simulink model "IntegratedBehaviorModule"  (R2024b)
settings: Solver=VariableStepAuto  StartTime=0.0  StopTime=inf  RelTol=1e-3
StartFcn:
  | clf
model workspace (MAT data in the model file):
  SL_ROS_VariableLengthArrays_MaxSizes.CommonInfo.ArrayTruncateAction = 'EmitWarning'
  SL_ROS_VariableLengthArrays_MaxSizes.MsgTypeMap = containers.Map
  SL_ROS_VariableLengthArrays_MaxSizes.MsgTypeMap.serialization.keys = {'std_msgs/Float32MultiArray', 'std_msgs/Float64MultiArray', 'std_msgs/Int8MultiArray'}
  SL_ROS_VariableLengthArrays_MaxSizes.MsgTypeMap.serialization.values{1}.PropertyName = 'data'
  SL_ROS_VariableLengthArrays_MaxSizes.MsgTypeMap.serialization.values{1}.DataType = 'single'
  SL_ROS_VariableLengthArrays_MaxSizes.MsgTypeMap.serialization.values{1}.MaxLength = 1500000
  SL_ROS_VariableLengthArrays_MaxSizes.MsgTypeMap.serialization.values{2}.PropertyName = 'data'
  SL_ROS_VariableLengthArrays_MaxSizes.MsgTypeMap.serialization.values{2}.DataType = 'double'
  SL_ROS_VariableLengthArrays_MaxSizes.MsgTypeMap.serialization.values{2}.MaxLength = 1500000
  SL_ROS_VariableLengthArrays_MaxSizes.MsgTypeMap.serialization.values{3}.PropertyName = 'data'
  SL_ROS_VariableLengthArrays_MaxSizes.MsgTypeMap.serialization.values{3}.DataType = 'int8'
  SL_ROS_VariableLengthArrays_MaxSizes.MsgTypeMap.serialization.values{3}.MaxLength = 1500000
  SL_ROS_VariableLengthArrays_MaxSizes.MsgTypeMap.serialization.uniformity = 0
  SL_ROS_VariableLengthArrays_MaxSizes.MsgTypeMap.serialization.keyType = 'char'
  SL_ROS_VariableLengthArrays_MaxSizes.MsgTypeMap.serialization.valueType = 'any'
  Sig = Simulink.Signal
  Sig.Dimensions = -1
  Sig.DimensionsMode = 'auto'
  Sig.Complexity = 'auto'
  Sig.SampleTime = -1
  Sig.SamplingMode = 'auto'
  Sig.DataType = 'auto'
undefined symbols (not defined in the file or in its folder): dem, fixedTEBParams, goalPose, initialTranslationTruck, mapSize, maxRefPathLen, nlobjTracking, pathBus_struct, TaskControllerModeType, tuneableTEBParamsCpp, tuneableTerrainAwareParams, worldGridLoc, worldMat, worldRes
libraries: simulink x10, roshelperlib x5, robotmobilelib x1, robotsim3dlib x1, sim3dlib x1
(part 1 of 2)
settings Model: DataDictionary=ros2lib.sldd  Creator=cstabile  LastModifiedBy=jbrault
settings SolverCC: DateTimeAtSimulationTimeZero=[]
settings OptimizationCC: BlockReduction=off  EnhancedBackFolding=on  PassReuseOutputArgsAs=Individual arguments  ZeroExternalMemoryAtStartup=off  ZeroInternalMemoryAtStartup=off  MaxStackSize=64  OptimizeBlockOrder=speed  DifferentSizesBufferReuse=on  OptimizationCustomize=off  EfficientTunableParamExpr=on
settings DebuggingCC: ParameterTunabilityLossMsg=error
settings ModelReferenceCC: UpdateModelReferenceTargets=IfOutOfDate
settings SFSimCC: SimTargetLang=C++
settings RTWCC: Description=Embedded Coder  SystemTargetFile=ert.tlc  HardwareBoard=Robot Operating System 2 (ROS 2)  TLCOptions="-aInlineSetEventsForThisBaseRateFcn=TLC_FALSE -aSuppressMultiTaskScheduler=TLC_FALSE  -aRateBasedStepFcn=0"  TemplateMakefile=ert_default_tmf  Toolchain=Colcon Tools  TargetLang=C++  GPUComputeCapability=3.5
settings CodeAppCC: ForceParamTrailComments=on  IgnoreCustomStorageClasses=off  OperatorAnnotations=on  SimulinkDataObjDesc=on  SFDataObjDesc=on  InsertBlockDesc=on
settings ERTTargetCC: CodeInterfacePackaging=C++ class  InlinedParameterPlacement=Hierarchical  RootIOFormat=Structure reference  DynamicArrayContainerType=coder::array

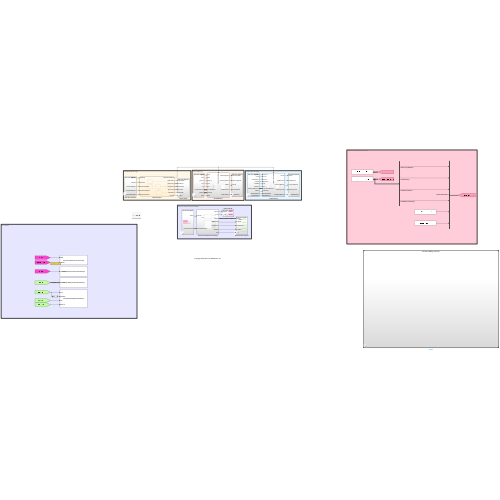
[thumbnail: Simulink's stored preview of the top-level diagram]
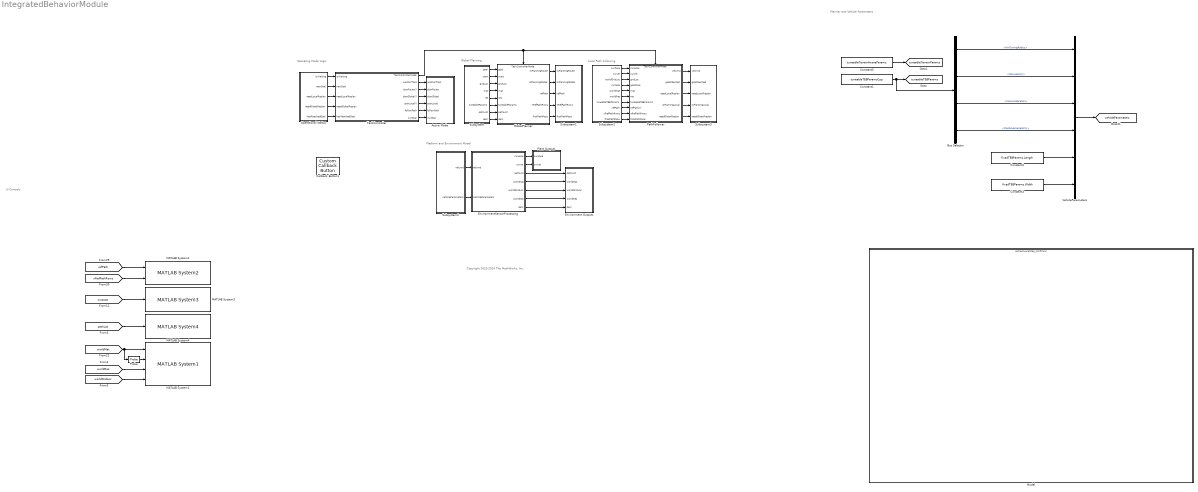
== system IntegratedBehaviorModule ==
  note: UI Controls
  note: Local Path Following
  note: Planner and Vehicle Parameters
  note: Global Planning
  note: Platform and Enviornment Model
  note: Operating Mode Logic
  note: Copyright 2023-2024 The MathWorks, Inc.
  Active Mode : Subsystem  Variant=on  VariantControl=Subsystem7
  Bus Selector : BusSelector  OutputSignals=MinTurningRadius,MaxVelocity,MaxAcceleration,MaxReverseVelocity
  Callback Button1 : CustomCallbackButton  Configuration="{\"components\":[{\"name\":\"BackgroundImageComponent\",\"settings\":{\"image\":{\"size\":[0,0],\"src\":\"default\",\"srcOrientation\":\"Right\"},\"position\":[0,0,1,1]}},{\"name\":\"ButtonStateComponent\",\"settings\":{\"buttonType\":\"momentary\",\"clickFcn\":\"set_param([bdroot(gcb) '\\/Operational Status\\/Simulink Signals\\/Confirm New Goal\\/newGoalBlock'],'Value','goalPose');\",\"onValue\":1,\"position\":[0,0,1,1],\"pressDelay\":\"500\",\"pressFcn\":\"\",\"repeatInterval\":\"0\",\"states\":[{\"horizontalAlignment\":\"center\",\"image\":{\"position\":[0,0,1,1],\"size\":[1,1],\"src\":\"default\",\"srcOrientation\":\"Right\"},\"label\":{\"color\":[0.01176470588,0.01176470588,0.01176470588,1],\"icon\":{\"size\":[0,0],\"src\":\"default\",\"srcOrientation\":\"Right\"},\"iconPlacement\":\"left\",\"opacity\":1,\"show\":true,\"text\":{\"content\":\"Update Goal\",\"font\":\"Helvetica\"}},\"labelOffset\":[0,0],\"verticalAlignment\":\"middle\"},{\"horizontalAlignment\":\"center\",\"image\":{\"position\":[0,0,1,1],\"size\":[1,1],\"src\":\"default\",\"srcOrientation\":\"Right\"},\"label\":{\"color\":[0.01176470588,0.01176470588,0.01176470588,1],\"icon\":{\"size\":[0,0],\"src\":\"default\",\"srcOrientation\":\"Right\"},\"iconPlacement\":\"left\",\"opacity\":1,\"show\":true,\"text\":{\"content\":\"Update Goal\",\"font\":\"Helvetica\"}},\"labelOffset\":[0,0],\"verticalAlignment\":\"middle\"},{\"horizontalAlignment\":\"center\",\"image\":{\"position\":[0,0,1,1],\"size\":[1,1],\"src\":\"default\",\"srcOrientation\":\"Right\"},\"label\":{\"color\":[0.01176470588,0.01176470588,0.01176470588,1],\"icon\":{\"size\":[0,0],\"src\":\"default\",\"srcOrientation\":\"Right\"},\"iconPlacement\":\"left\",\"opacity\":1,\"show\":true,\"text\":{\"content\":\"Update Goal\",\"font\":\"Helvetica\"}},\"labelOffset\":[0,0],\"verticalAlignment\":\"middle\"},{\"horizontalAlignment\":\"center\",\"image\":{\"position\":[0,0,1,1],\"size\":[1,1],\"src\":\"default\",\"srcOrientation\":\"Right\"},\"label\":{\"color\":[0.01176470588,0.01176470588,0.01176470588,1],\"icon\":{\"size\":[0,0],\"src\":\"default\",\"srcOrientation\":\"Right\"},\"iconPlacement\":\"left\",\"opacity\":1,\"show\":true,\"text\":{\"content\":\"Update Goal\",\"font\":\"Helvetica\"}},\"labelOffset\":[0,0],\"verticalAlignment\":\"middle\"}]}},{\"name\":\"ForegroundImageComponent\",\"settings\":{\"image\":{\"size\":[0,0],\"src\":\"default\",\"srcOrientation\":\"Right\"},\"isForeground\":1,\"position\":[0,0,1,1]}}],\"settings\":{\"BindingType\":\"standalone\",\"backgroundColor\":[244,244,244,1],\"backgroundOffset\":0.2,\"backgroundOpacity\":1,\"fixedAspectRatio\":\"off\",\"foregroundColor\":[0.01176470588,0.01176470588,0.01176470588,1],\"migratedFromLegacy\":true,\"useBackgroundColor\":true,\"variant\":\"callback\",\"version\":\"R2024b\"},\"type\":\"Button\"}"  CustomBackgroundColor="{\"color\":[0.9568627451,0.9568627451,0.9568627451],\"show\":true}"
  Constant1 : Constant  Value=tuneableTEBParamsCpp  VectorParams1D=off  OutDataTypeStr=Bus: teb_bus
  Constant2 : Constant  Value=fixedTEBParams.Length  VectorParams1D=off
  Constant3 : Constant  Value=fixedTEBParams.Width  VectorParams1D=off
  Constant5 : Constant  Value=tuneableTerrainAwareParams  VectorParams1D=off  OutDataTypeStr=Bus: fsp_tunable_bus
  Environment Outputs : Subsystem  Variant=on  VariantControl=Subsystem6
  EnvironmentSensorProcessing : Subsystem
  GlobalPlanner : Subsystem
      settings: PortSchema="{\"entries\":[{\"content\":{\"sides\":[{\"content\":{\"connectorIds\":[\"In1\",\"In2\",\"In3\",\"In4\",\"In5\",\"In6\",\"In7\",\"In8\"]},\"type\":\"ConnectorPlacement.EquallySpacedRectSide\",\"uuid\":\"aee3cac8-8097-4690-922a-bc1b3519889f\"},{\"content\":{\"connectorIds\":[\"Out1\",\"Out2\",\"Out3\",\"Out4\",\"Out5\"],\"side\":\"RIGHT\"},\"type\":\"ConnectorPlacement.EquallySpacedRectSide\",\"uuid\":\"5687e6bb-e602-4583-a132-0948be564698\"},{\"content\":{\"connectorIds\":[\"In9\"],\"side\":\"TOP\"},\"type\":\"ConnectorPlacement.EquallySpacedRectSide\",\"uuid\":\"0e247324-6f1c-4085-8c8a-e90842b5aeca\"}]},\"type\":\"ConnectorPlacement.EquallySpacedConnector\",\"uuid\":\"2bd2942a-c08c-4913-ac88-5c0c00cdacfd\"}],\"packageUris\":[\"http://schema.mathworks.com/mf0/Connector/R2020b\"],\"version\":\"1.0\"}"
  MATLAB System1 : roshelperlib/MATLAB System1  MapType=Bin  IsEgo=off  DisplayVisual=on  SimulateUsing=Interpreted execution
  MATLAB System2 : roshelperlib/MATLAB System2  VisualizationParameters={'Color','#D95319','LineWidth',3}  PlotType=Line  DisplayVisual=on  SimulateUsing=Interpreted execution
  MATLAB System3 : roshelperlib/MATLAB System3  NumCircles=3  Length=fixedTEBParams.Length  Width=fixedTEBParams.Width  DisplayVisual=on  SimulateUsing=Interpreted execution
  MATLAB System4 : roshelperlib/MATLAB System4  NodeColor=#0072BD  EdgeColor=#0072BD  LineStyle=-  GraphSpec=cell(1,0)  NetworkColor=#0072BD  NetworkStyle=:  NetworkSpec=cell(1,0)  MaxEdgeElem=maxElementPerEdge  NetworkAlpha=.25  EdgeAlpha=0  DisplayVisual=on  SimulateUsing=Interpreted execution
  Model : ModelReference  ModelNameDialog=extractLocalMap_simfcnsvr.slx  SimulationMode=Normal  ScheduleRates=on  ModelReferenceVersion=1.4
  Operational Status : Subsystem  Variant=on  VariantControl=Subsystem8
  PathFollower : Subsystem
      settings: PortSchema="{\"entries\":[{\"content\":{\"sides\":[{\"content\":{\"connectorIds\":[\"In1\",\"In2\",\"In3\",\"In4\",\"In5\",\"In6\",\"In7\",\"In8\",\"In9\",\"In10\"]},\"type\":\"ConnectorPlacement.EquallySpacedRectSide\",\"uuid\":\"7812fcae-0375-4e84-8c7b-4e703c496332\"},{\"content\":{\"connectorIds\":[\"Out1\",\"Out2\",\"Out3\",\"Out4\",\"Out5\"],\"side\":\"RIGHT\"},\"type\":\"ConnectorPlacement.EquallySpacedRectSide\",\"uuid\":\"b2008f15-9cd5-4726-942a-198ff51360c1\"},{\"content\":{\"connectorIds\":[\"In11\"],\"side\":\"TOP\"},\"type\":\"ConnectorPlacement.EquallySpacedRectSide\",\"uuid\":\"7bcf1b97-5d60-48cd-a54d-4c6f1d8d04a5\"}]},\"type\":\"ConnectorPlacement.EquallySpacedConnector\",\"uuid\":\"0b288f00-763d-4136-89b5-29e3b1e07301\"}],\"packageUris\":[\"http://schema.mathworks.com/mf0/Connector/R2020b\"],\"version\":\"1.0\"}"
  Plant Outputs : Subsystem  Variant=on  VariantControl=Subsystem5
  Probe : Probe  ProbeWidth=off  ProbeSampleTime=off  ProbeComplexSignal=off  ProbeSignalDimensions=on
  Subsystem : Subsystem  Variant=on  VariantControl=Subsystem
  Subsystem1 : Subsystem  Variant=on  VariantControl=Subsystem1
  Subsystem2 : Subsystem  Variant=on  VariantControl=Subsystem2
  Subsystem3 : Subsystem  Variant=on  VariantControl=Subsystem3
  Subsystem4 : Subsystem  Variant=on  VariantControl=Subsystem4
  TaskController : Stateflow chart  TreatAsAtomicUnit=on
      settings: PortSchema="{\"entries\":[{\"content\":{\"sides\":[{\"content\":{\"connectorIds\":[\"In1\",\"In2\",\"In4\",\"In3\",\"In5\"]},\"type\":\"ConnectorPlacement.EquallySpacedRectSide\",\"uuid\":\"cbfa7659-89a5-4e0b-94c8-c3ff629b6c07\"},{\"content\":{\"connectorIds\":[\"Out4\",\"Out1\",\"Out6\",\"Out7\",\"Out5\",\"Out2\",\"Out3\"],\"side\":\"RIGHT\"},\"type\":\"ConnectorPlacement.EquallySpacedRectSide\",\"uuid\":\"09a77d14-4924-404f-bc0a-d1cd3933e1ef\"},{\"content\":{\"side\":\"TOP\"},\"type\":\"ConnectorPlacement.EquallySpacedRectSide\",\"uuid\":\"bb1c4e19-123f-41f1-a220-47cc74084463\"}]},\"type\":\"ConnectorPlacement.EquallySpacedConnector\",\"uuid\":\"cd7ce687-884d-40d4-a1d1-e5ac9833bd00\"}],\"packageUris\":[\"http://schema.mathworks.com/mf0/Connector/R2020b\"],\"version\":\"1.0\"}"
  VehicleParameters : BusCreator  Inputs=6
  tag scope: tuneableTEBParams=global, tuneableTerrainParams=global, vehicleParameters=global
  wires:
  Constant1/1 -> [tuneableTEBParams], Bus Selector/1
  Constant5/1 -> [tuneableTerrainParams]
  Bus Selector/1 -> VehicleParameters/1  "<MinTurningRadius>"
  Bus Selector/2 -> VehicleParameters/2  "<MaxVelocity>"
  Constant3/1 -> VehicleParameters/6
  Constant2/1 -> VehicleParameters/5
  Bus Selector/3 -> VehicleParameters/3  "<MaxAcceleration>"
  Bus Selector/4 -> VehicleParameters/4  "<MaxReverseVelocity>"
  VehicleParameters/1 -> [vehicleParameters]
  Subsystem/1(goal) -> GlobalPlanner/1(goal)
  Subsystem/2(start) -> GlobalPlanner/2(start)
  Subsystem/3(gridLoc) -> GlobalPlanner/3(gridLoc)
  Subsystem/4(mat) -> GlobalPlanner/4(mat)
  Subsystem/5(res) -> GlobalPlanner/5(res)
  Subsystem/6(tuneableParams) -> GlobalPlanner/6(tuneableParams)
  Subsystem/7(pathList) -> GlobalPlanner/7(pathList)
  Subsystem/8(dem) -> GlobalPlanner/8(dem)
  GlobalPlanner/1(isPlanningRoute) -> Subsystem1/1(isPlanningRoute)
  GlobalPlanner/2(isPlanningGlobal) -> Subsystem1/2(isPlanningGlobal)
  GlobalPlanner/3(refPath) -> Subsystem1/3(refPath)
  GlobalPlanner/4(nRefPathRows) -> Subsystem1/4(nRefPathRows)
  GlobalPlanner/5(finalPathPose) -> Subsystem1/5(finalPathPose)
  Subsystem2/1(curPose) -> PathFollower/1(curpose)
  Subsystem2/2(curvel) -> PathFollower/2(curvel)
  Subsystem2/3(worldGridLoc) -> PathFollower/3(gridLoc)
  Subsystem2/4(curGoal) -> PathFollower/4(goalPose)
  Subsystem2/5(worldMat) -> PathFollower/5(mat)
  Subsystem2/6(worldRes) -> PathFollower/6(res)
  Subsystem2/7(tuneableTEBParams) -> PathFollower/7(tuneableTEBParams)
  Subsystem2/8(refPath) -> PathFollower/8(refPathXY)
  Subsystem2/9(nRefPathRows) -> PathFollower/9(nRefPathRows)
  Subsystem2/10(finalPathPose) -> PathFollower/10(finalPathPose)
  PathFollower/1(velcmd) -> Subsystem3/1(velcmd)
  PathFollower/2(goalReached) -> Subsystem3/2(goalReached)
  PathFollower/3(needLocalReplan) -> Subsystem3/3(needLocalReplan)
  PathFollower/4(isPlanningLocal) -> Subsystem3/4(isPlanningLocal)
  PathFollower/5(needGlobalReplan) -> Subsystem3/5(needGlobalReplan)
  Subsystem4/1(velcmd) -> EnvironmentSensorProcessing/1(velcmd)
  Subsystem4/2(vehicleParameters) -> EnvironmentSensorProcessing/2(VehicleParameters)
  EnvironmentSensorProcessing/1(curpose) -> Plant Outputs/1(curpose)
  EnvironmentSensorProcessing/2(curvel) -> Plant Outputs/2(curvel)
  EnvironmentSensorProcessing/3(pathList) -> Environment Outputs/1(pathList)
  EnvironmentSensorProcessing/4(worldMat) -> Environment Outputs/2(worldMat)
  EnvironmentSensorProcessing/5(worldGridLoc) -> Environment Outputs/3(worldGridLoc)
  EnvironmentSensorProcessing/6(worldRes) -> Environment Outputs/4(worldRes)
  EnvironmentSensorProcessing/7(dem) -> Environment Outputs/5(dem)
  TaskController/1(waitForTask) -> Active Mode/1(waitForTask)
  TaskController/3(curGoal) -> Active Mode/6(curGoal)
  TaskController/6(planRoute()) -> Active Mode/2(planRoute)
  TaskController/2(followPath) -> Active Mode/5(followPath)
  Probe/1 -> MATLAB System1/2
  TaskController/5(planLocal()) -> Active Mode/4(planLocal)
  TaskController/7(planGlobal()) -> Active Mode/3(planGlobal)
  [worldMat] -> MATLAB System1/1, Probe/1
  [pathList] -> MATLAB System4/1
  [curpose] -> MATLAB System3/1
  [worldRes] -> MATLAB System1/3
  [worldGridLoc] -> MATLAB System1/4
  [refPath] -> MATLAB System2/1
  [nRefPathRows] -> MATLAB System2/2
  Operational Status/4(needGlobalReplan) -> TaskController/3(needGlobalReplan)
  Operational Status/5(hasReachedGoal) -> TaskController/5(hasReachedGoal)
  Operational Status/3(needLocalReplan) -> TaskController/4(needLocalReplan)
  TaskController/4(TaskControllerMode) -> PathFollower/11(TaskControllerMode), GlobalPlanner/9(TaskControllerMode)
  Operational Status/1(isWaiting) -> TaskController/1(isWaiting)
  Operational Status/2(newGoal) -> TaskController/2(newGoal)

== system IntegratedBehaviorModule/Active Mode ==
  waitForTask : Inport
  planRoute : Inport  Port=2
  planGlobal : Inport  Port=3
  planLocal : Inport  Port=4
  followPath : Inport  Port=5
  curGoal : Inport  Port=6
  Simulink Signals : Subsystem  VariantControl="vssCommProtocol == \"SLSignals\""

== system IntegratedBehaviorModule/Environment Outputs ==
  pathList : Inport
  worldMat : Inport  Port=2
  worldGridLoc : Inport  Port=3
  worldRes : Inport  Port=4
  dem : Inport  Port=5
  Simulink Signals : Subsystem  VariantControl="vssCommProtocol == \"SLSignals\""

== system IntegratedBehaviorModule/EnvironmentSensorProcessing ==
  velcmd : Inport
  VehicleParameters : Inport  Port=2
  Environment State : Subsystem
  Platform Model : Subsystem  Variant=on  VariantControl=Environemnt
  curpose : Outport
  curvel : Outport  Port=2
  pathList : Outport  Port=3
  worldMat : Outport  Port=4
  worldGridLoc : Outport  Port=5
  worldRes : Outport  Port=6
  dem : Outport  Port=7
  wires:
  Environment State/1(pathList) -> pathList/1
  Environment State/2(worldMat) -> worldMat/1
  Environment State/3(worldGridLoc) -> worldGridLoc/1
  Environment State/4(worldRes) -> worldRes/1
  Environment State/5(dem) -> dem/1
  velcmd/1 -> Platform Model/1(velcmd)
  VehicleParameters/1 -> Platform Model/2(VehicleParameters)
  Platform Model/1(curpose) -> curpose/1
  Platform Model/2(curvel) -> curvel/1

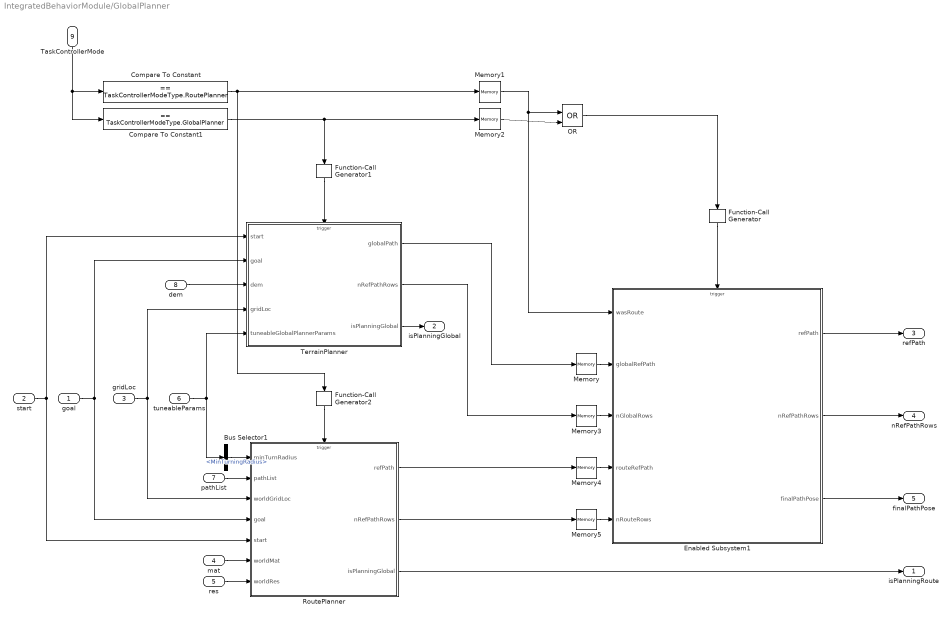
== system IntegratedBehaviorModule/GlobalPlanner ==
  goal : Inport
  start : Inport  Port=2
  gridLoc : Inport  Port=3
  mat : Inport  Port=4
  res : Inport  Port=5
  tuneableParams : Inport  Port=6
  pathList : Inport  Port=7
  dem : Inport  Port=8
  TaskControllerMode : Inport  Port=9
  Bus Selector1 : BusSelector  OutputSignals=MinTurningRadius
  Compare To Constant : simulink/Logic and Bit Operations/Compare To Constant  relop===  const=TaskControllerModeType.RoutePlanner  OutDataTypeStr=boolean
  Compare To Constant1 : simulink/Logic and Bit Operations/Compare To Constant  relop===  const=TaskControllerModeType.GlobalPlanner  OutDataTypeStr=boolean
  Enabled Subsystem1 : Subsystem  TreatAsAtomicUnit=on
  Function-Call Generator : simulink/Ports & Subsystems/Function-Call Generator  sample_time=1  numberOfIterations=1  DisallowWideOutput=off  ShowEnablePort=on
  Function-Call Generator1 : simulink/Ports & Subsystems/Function-Call Generator  sample_time=1  numberOfIterations=1  DisallowWideOutput=off  ShowEnablePort=on
  Function-Call Generator2 : simulink/Ports & Subsystems/Function-Call Generator  sample_time=1  numberOfIterations=1  DisallowWideOutput=off  ShowEnablePort=on
  Memory{,1..5} (6 alike) : Memory
  OR : Logic  Operator=OR  IconShape=distinctive  AllPortsSameDT=off  OutDataTypeStr=boolean
  RoutePlanner : Subsystem
  TerrainPlanner : Subsystem
  isPlanningRoute : Outport
  isPlanningGlobal : Outport  Port=2
  refPath : Outport  Port=3
  nRefPathRows : Outport  Port=4
  finalPathPose : Outport  Port=5
  wires:
  start/1 -> RoutePlanner/5(start), TerrainPlanner/1(start)
  RoutePlanner/1(refPath) -> Memory4/1
  pathList/1 -> RoutePlanner/2(pathList)
  Enabled Subsystem1/2(nRefPathRows) -> nRefPathRows/1
  TerrainPlanner/2(nRefPathRows) -> Memory3/1
  mat/1 -> RoutePlanner/6(worldMat)
  res/1 -> RoutePlanner/7(worldRes)
  Enabled Subsystem1/1(refPath) -> refPath/1
  tuneableParams/1 -> Bus Selector1/1, TerrainPlanner/5(tuneableGlobalPlannerParams)
  goal/1 -> RoutePlanner/4(goal), TerrainPlanner/2(goal)
  dem/1 -> TerrainPlanner/3(dem)
  RoutePlanner/3(isPlanningGlobal) -> isPlanningRoute/1
  RoutePlanner/2(nRefPathRows) -> Memory5/1
  TerrainPlanner/1(globalPath) -> Memory/1
  gridLoc/1 -> TerrainPlanner/4(gridLoc), RoutePlanner/3(worldGridLoc)
  Enabled Subsystem1/3(finalPathPose) -> finalPathPose/1
  Bus Selector1/1 -> RoutePlanner/1(minTurnRadius)  "<MinTurningRadius>"
  TerrainPlanner/3(isPlanningGlobal) -> isPlanningGlobal/1
  Compare To Constant/1 -> Memory1/1, Function-Call Generator2/1
  Function-Call Generator1/1 -> TerrainPlanner/Trigger
  Function-Call Generator2/1 -> RoutePlanner/Trigger
  Compare To Constant1/1 -> Memory2/1, Function-Call Generator1/1
  Function-Call Generator/1 -> Enabled Subsystem1/Trigger
  OR/1 -> Function-Call Generator/1
  TaskControllerMode/1 -> Compare To Constant/1, Compare To Constant1/1
  Memory1/1 -> OR/1, Enabled Subsystem1/1(wasRoute)
  Memory2/1 -> OR/2
  Memory/1 -> Enabled Subsystem1/2(globalRefPath)
  Memory3/1 -> Enabled Subsystem1/3(nGlobalRows)
  Memory4/1 -> Enabled Subsystem1/4(routeRefPath)
  Memory5/1 -> Enabled Subsystem1/5(nRouteRows)

== system IntegratedBehaviorModule/Operational Status ==
  Simulink Signals : Subsystem  VariantControl="vssCommProtocol == \"SLSignals\""
  isWaiting : Outport
  newGoal : Outport  Port=2
  needLocalReplan : Outport  Port=3
  needGlobalReplan : Outport  Port=4
  hasReachedGoal : Outport  Port=5

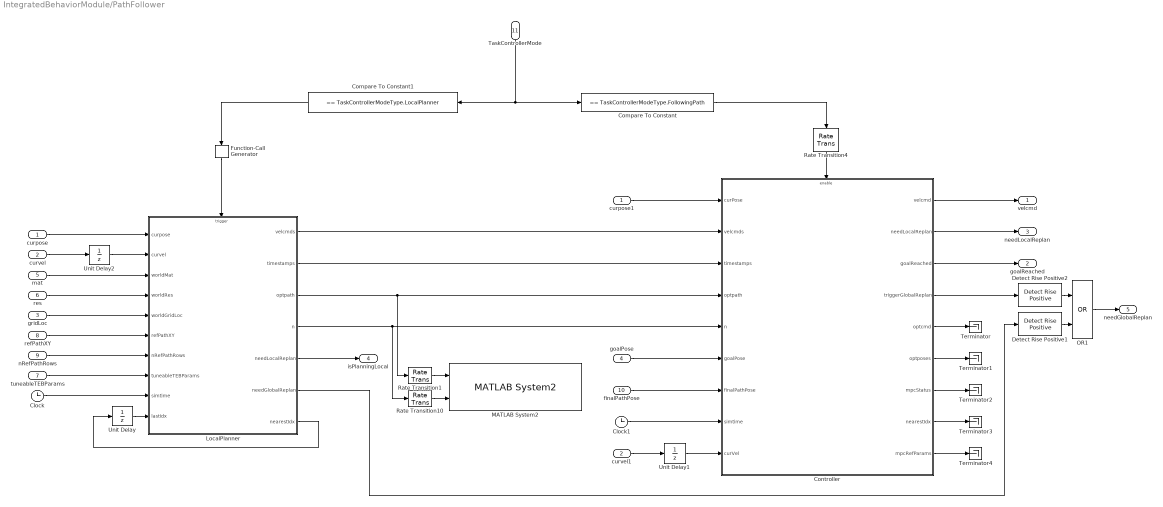
== system IntegratedBehaviorModule/PathFollower ==
  curpose : Inport  PortDimensions=[1 3]
  curvel : Inport  Port=2  PortDimensions=[1 2]
  gridLoc : Inport  Port=3
  goalPose : Inport  Port=4
  mat : Inport  Port=5
  res : Inport  Port=6
  tuneableTEBParams : Inport  Port=7
  refPathXY : Inport  Port=8
  nRefPathRows : Inport  Port=9
  finalPathPose : Inport  Port=10
  TaskControllerMode : Inport  Port=11
  Clock : Clock
  Clock1 : Clock
  Compare To Constant : simulink/Logic and Bit Operations/Compare To Constant  relop===  const=TaskControllerModeType.FollowingPath  OutDataTypeStr=boolean
  Compare To Constant1 : simulink/Logic and Bit Operations/Compare To Constant  relop===  const=TaskControllerModeType.LocalPlanner  OutDataTypeStr=boolean
  Controller : Subsystem  Variant=on  VariantControlMode=label  VariantControl=Controller  LabelModeActiveChoice=TEB MPC Cascade
  Detect Rise Positive1 : simulink/Logic and Bit Operations/Detect Rise Positive  vinit=0  OutDataTypeStr=boolean
  Detect Rise Positive2 : simulink/Logic and Bit Operations/Detect Rise Positive  vinit=0  OutDataTypeStr=boolean
  Function-Call Generator : simulink/Ports & Subsystems/Function-Call Generator  sample_time=1  numberOfIterations=1  DisallowWideOutput=off  ShowEnablePort=on
  LocalPlanner : Subsystem
  MATLAB System2 : roshelperlib/MATLAB System2  VisualizationParameters={'c:','LineWidth',3}  PlotType=Line  DisplayVisual=on  SimulateUsing=Interpreted execution
  OR1 : Logic  Operator=OR  IconShape=distinctive  AllPortsSameDT=off  OutDataTypeStr=boolean
  Rate Transition1 : RateTransition  OutPortSampleTime=nlobjTracking.Ts
  Rate Transition10 : RateTransition  OutPortSampleTime=nlobjTracking.Ts
  Rate Transition4 : RateTransition  OutPortSampleTime=nlobjTracking.Ts
  Terminator{,1..4} (5 alike) : Terminator
  Unit Delay : UnitDelay  InitialCondition=1  SampleTime=-1  HasFrameUpgradeWarning=on
  Unit Delay1 : UnitDelay  SampleTime=-1  HasFrameUpgradeWarning=on
  Unit Delay2 : UnitDelay  SampleTime=-1  HasFrameUpgradeWarning=on
  curpose1 : InportShadow  PortDimensions=[1 3]
  curvel1 : InportShadow  Port=2  PortDimensions=[1 2]
  velcmd : Outport
  goalReached : Outport  Port=2
  needLocalReplan : Outport  Port=3
  isPlanningLocal : Outport  Port=4
  needGlobalReplan : Outport  Port=5
  wires:
  refPathXY/1 -> LocalPlanner/6(refPathXY)
  gridLoc/1 -> LocalPlanner/5(worldGridLoc)
  mat/1 -> LocalPlanner/3(worldMat)
  res/1 -> LocalPlanner/4(worldRes)
  nRefPathRows/1 -> LocalPlanner/7(nRefPathRows)
  tuneableTEBParams/1 -> LocalPlanner/8(tuneableTEBParams)
  Clock/1 -> LocalPlanner/9(simtime)
  LocalPlanner/5(needLocalReplan) -> isPlanningLocal/1
  Function-Call Generator/1 -> LocalPlanner/Trigger
  Controller/1(velcmd) -> velcmd/1
  Controller/2(needLocalReplan) -> needLocalReplan/1
  Controller/3(goalReached) -> goalReached/1
  Controller/5(optcmd) -> Terminator/1
  Controller/7(mpcStatus) -> Terminator2/1
  Controller/8(nearestIdx) -> Terminator3/1
  Controller/9(mpcRefParams) -> Terminator4/1
  Controller/6(optposes) -> Terminator1/1
  Controller/4(triggerGlobalReplan) -> Detect Rise Positive2/1
  LocalPlanner/6(needGlobalReplan) -> Detect Rise Positive1/1
  OR1/1 -> needGlobalReplan/1
  Detect Rise Positive1/1 -> OR1/2
  Detect Rise Positive2/1 -> OR1/1
  curpose/1 -> LocalPlanner/1(curpose)
  curvel/1 -> Unit Delay2/1
  LocalPlanner/7(nearestIdx) -> Unit Delay/1
  Unit Delay/1 -> LocalPlanner/10(lastIdx)
  Rate Transition1/1 -> MATLAB System2/1
  Rate Transition10/1 -> MATLAB System2/2
  LocalPlanner/1(velcmds) -> Controller/2(velcmds)
  LocalPlanner/2(timestamps) -> Controller/3(timestamps)
  LocalPlanner/3(optpath) -> Rate Transition1/1, Controller/4(optpath)
  LocalPlanner/4(n) -> Rate Transition10/1, Controller/5(n)
  goalPose/1 -> Controller/6(goalPose)
  finalPathPose/1 -> Controller/7(finalPathPose)
  Clock1/1 -> Controller/8(simtime)
  Rate Transition4/1 -> Controller/Enable
  curvel1/1 -> Unit Delay1/1
  curpose1/1 -> Controller/1(curPose)
  TaskControllerMode/1 -> Compare To Constant1/1, Compare To Constant/1
  Compare To Constant/1 -> Rate Transition4/1
  Compare To Constant1/1 -> Function-Call Generator/1
  Unit Delay1/1 -> Controller/9(curVel)
  Unit Delay2/1 -> LocalPlanner/2(curvel)

== system IntegratedBehaviorModule/Plant Outputs ==
  curpose : Inport
  curvel : Inport  Port=2
  Simulink Signals : Subsystem  VariantControl="vssCommProtocol == \"SLSignals\""

== system IntegratedBehaviorModule/Subsystem ==
  Simulink Signals : Subsystem  VariantControl="vssCommProtocol == \"SLSignals\""
  goal : Outport
  start : Outport  Port=2
  gridLoc : Outport  Port=3
  mat : Outport  Port=4
  res : Outport  Port=5
  tuneableParams : Outport  Port=6
  pathList : Outport  Port=7
  dem : Outport  Port=8

== system IntegratedBehaviorModule/Subsystem1 ==
  isPlanningRoute : Inport
  isPlanningGlobal : Inport  Port=2
  refPath : Inport  Port=3
  nRefPathRows : Inport  Port=4
  finalPathPose : Inport  Port=5
  Simulink Signals : Subsystem  VariantControl="vssCommProtocol == \"SLSignals\""

== system IntegratedBehaviorModule/Subsystem2 ==
  Simulink Signals : Subsystem  VariantControl="vssCommProtocol == \"SLSignals\""
  curPose : Outport
  curvel : Outport  Port=2
  worldGridLoc : Outport  Port=3
  curGoal : Outport  Port=4
  worldMat : Outport  Port=5
  worldRes : Outport  Port=6
  tuneableTEBParams : Outport  Port=7
  refPath : Outport  Port=8
  nRefPathRows : Outport  Port=9
  finalPathPose : Outport  Port=10

== system IntegratedBehaviorModule/Subsystem3 ==
  velcmd : Inport
  goalReached : Inport  Port=2
  needLocalReplan : Inport  Port=3
  isPlanningLocal : Inport  Port=4
  needGlobalReplan : Inport  Port=5
  Simulink Signals : Subsystem  VariantControl="vssCommProtocol == \"SLSignals\""

== system IntegratedBehaviorModule/Subsystem4 ==
  Simulink Signals : Subsystem  VariantControl="vssCommProtocol == \"SLSignals\""
  velcmd : Outport
  vehicleParameters : Outport  Port=2

== system IntegratedBehaviorModule/Active Mode/Simulink Signals ==
  waitForTask : Inport
  planRoute : Inport  Port=2
  planGlobal : Inport  Port=3
  planLocal : Inport  Port=4
  followPath : Inport  Port=5
  curGoal : Inport  Port=6
  tag scope: curGoal=global, followPath=global, planGlobal=global, planLocal=global, planRoute=global, waitForTask=global
  wires:
  followPath/1 -> [followPath]
  planGlobal/1 -> [planGlobal]
  waitForTask/1 -> [waitForTask]
  planRoute/1 -> [planRoute]
  planLocal/1 -> [planLocal]
  curGoal/1 -> [curGoal]

== system IntegratedBehaviorModule/Environment Outputs/Simulink Signals ==
  pathList : Inport
  worldMat : Inport  Port=2
  worldGridLoc : Inport  Port=3
  worldRes : Inport  Port=4
  dem : Inport  Port=5
  tag scope: dem=global, pathList=global, worldGridLoc=global, worldMat=global, worldRes=global
  wires:
  worldGridLoc/1 -> [worldGridLoc]
  pathList/1 -> [pathList]
  dem/1 -> [dem]
  worldMat/1 -> [worldMat]
  worldRes/1 -> [worldRes]

== system IntegratedBehaviorModule/EnvironmentSensorProcessing/Environment State ==
  note: Environment State
  Constant : Constant  Value=worldMat  VectorParams1D=off
  Constant2 : Constant  Value=pathBus_struct  VectorParams1D=off  OutDataTypeStr=Bus: pathList_fixed_bus
  Constant4 : Constant  Value=dem  VectorParams1D=off
  gridLoc : Constant  Value=worldGridLoc  VectorParams1D=off
  res : Constant  Value=worldRes
  pathList : Outport
  worldMat : Outport  Port=2
  worldGridLoc : Outport  Port=3
  worldRes : Outport  Port=4
  dem : Outport  Port=5
  wires:
  Constant2/1 -> pathList/1
  Constant4/1 -> dem/1
  Constant/1 -> worldMat/1
  gridLoc/1 -> worldGridLoc/1
  res/1 -> worldRes/1

== system IntegratedBehaviorModule/EnvironmentSensorProcessing/Platform Model ==
  velcmd : Inport
  VehicleParameters : Inport  Port=2
  Bicycle Model (2D) : Subsystem  VariantControl="vssPhysModel == \"Simple\""
  Unreal (3D) : Subsystem  VariantControl="vssPhysModel == \"Unreal\""
  curpose : Outport
  curvel : Outport  Port=2

== system IntegratedBehaviorModule/GlobalPlanner/Enabled Subsystem1 ==
  wasRoute : Inport
  globalRefPath : Inport  Port=2
  nGlobalRows : Inport  Port=3
  routeRefPath : Inport  Port=4
  nRouteRows : Inport  Port=5
  Trigger : TriggerPort  TriggerType=function-call  VariantControl=(inherit)  PortDimensions=1
  Selector : Selector  NumberOfDimensions=2  InputPortWidth=1  IndexOptions=Index vector (port),Select all  Indices=[1 3],1  OutputSizes=1,1
  Switch : Switch  Criteria=u2 > Threshold  SaturateOnIntegerOverflow=off  InputSameDT=off
  Switch1 : Switch  Criteria=u2 > Threshold  SaturateOnIntegerOverflow=off  InputSameDT=off
  refPath : Outport
  nRefPathRows : Outport  Port=2
  finalPathPose : Outport  Port=3
  wires:
  wasRoute/1 -> Switch1/2, Switch/2
  globalRefPath/1 -> Switch/3
  routeRefPath/1 -> Switch/1
  nRouteRows/1 -> Switch1/1
  nGlobalRows/1 -> Switch1/3
  Switch/1 -> Selector/1, refPath/1
  Selector/1 -> finalPathPose/1
  Switch1/1 -> Selector/2, nRefPathRows/1

== system IntegratedBehaviorModule/GlobalPlanner/RoutePlanner ==
  minTurnRadius : Inport
  pathList : Inport  Port=2
  worldGridLoc : Inport  Port=3
  goal : Inport  Port=4
  start : Inport  Port=5
  worldMat : Inport  Port=6
  worldRes : Inport  Port=7
  planRoute : TriggerPort  TriggerType=function-call  VariantControl=(inherit)  PortDimensions=1
  Constant : Constant  Value=0
  Function Caller : FunctionCaller  FunctionPrototype=[refPath,nRefPathRows] = planRoute(pathList,start,goal,worldMat,gridLoc,res,minTurnRadius)  InputArgumentSpecifications=<Enter example>  OutputArgumentSpecifications=<Enter example>
  refPath : Outport
  nRefPathRows : Outport  Port=2
  isPlanningGlobal : Outport  Port=3
  wires:
  minTurnRadius/1 -> Function Caller/7
  start/1 -> Function Caller/2
  worldRes/1 -> Function Caller/6
  worldMat/1 -> Function Caller/4
  pathList/1 -> Function Caller/1
  worldGridLoc/1 -> Function Caller/5
  goal/1 -> Function Caller/3
  Function Caller/1 -> refPath/1
  Function Caller/2 -> nRefPathRows/1
  Constant/1 -> isPlanningGlobal/1

== system IntegratedBehaviorModule/GlobalPlanner/TerrainPlanner ==
  start : Inport
  goal : Inport  Port=2
  dem : Inport  Port=3
  gridLoc : Inport  Port=4
  tuneableGlobalPlannerParams : Inport  Port=5
  planGlobal : TriggerPort  TriggerType=function-call  VariantControl=(inherit)  PortDimensions=1
  Constant : Constant  Value=0
  Function Caller : FunctionCaller  FunctionPrototype=[globalPath,nRefPathRows] = planGlobal(start,goal,dem,gridLoc,tuneableGlobalPlannerParams)  InputArgumentSpecifications=<Enter example>  OutputArgumentSpecifications=<Enter example>
  globalPath : Outport
  nRefPathRows : Outport  Port=2
  isPlanningGlobal : Outport  Port=3
  wires:
  tuneableGlobalPlannerParams/1 -> Function Caller/5
  dem/1 -> Function Caller/3
  start/1 -> Function Caller/1
  Function Caller/1 -> globalPath/1
  Function Caller/2 -> nRefPathRows/1
  gridLoc/1 -> Function Caller/4
  goal/1 -> Function Caller/2
  Constant/1 -> isPlanningGlobal/1

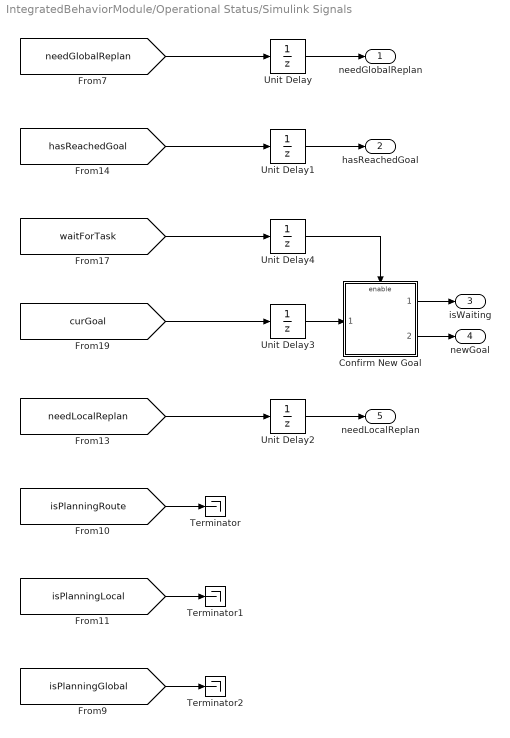
== system IntegratedBehaviorModule/Operational Status/Simulink Signals ==
  Confirm New Goal : Subsystem  TreatAsAtomicUnit=on
  Terminator : Terminator
  Terminator1 : Terminator
  Terminator2 : Terminator
  Unit Delay{,1..4} (5 alike) : UnitDelay  SampleTime=-1  HasFrameUpgradeWarning=on
  needGlobalReplan : Outport
  hasReachedGoal : Outport  Port=2
  isWaiting : Outport  Port=3
  newGoal : Outport  Port=4
  needLocalReplan : Outport  Port=5
  wires:
  [needGlobalReplan] -> Unit Delay/1
  [hasReachedGoal] -> Unit Delay1/1
  [waitForTask] -> Unit Delay4/1
  [curGoal] -> Unit Delay3/1
  [needLocalReplan] -> Unit Delay2/1
  Unit Delay4/1 -> Confirm New Goal/Enable
  Unit Delay3/1 -> Confirm New Goal/1(curGoal)
  Unit Delay2/1 -> needLocalReplan/1
  [isPlanningRoute] -> Terminator/1
  [isPlanningLocal] -> Terminator1/1
  [isPlanningGlobal] -> Terminator2/1
  Unit Delay/1 -> needGlobalReplan/1
  Unit Delay1/1 -> hasReachedGoal/1
  Confirm New Goal/1(isWaiting) -> isWaiting/1
  Confirm New Goal/2(newGoal) -> newGoal/1

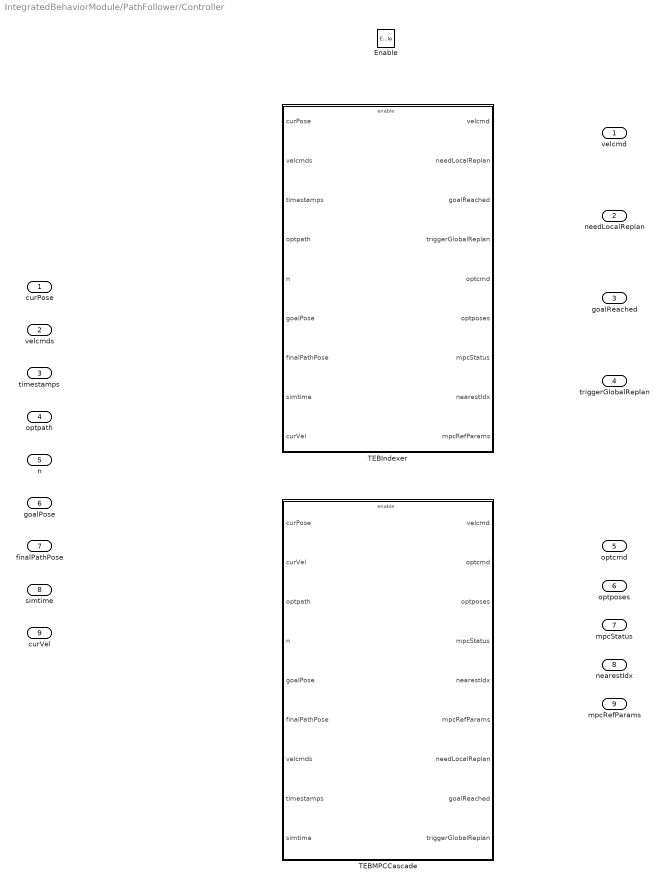
== system IntegratedBehaviorModule/PathFollower/Controller ==
  curPose : Inport
  velcmds : Inport  Port=2
  timestamps : Inport  Port=3
  optpath : Inport  Port=4
  n : Inport  Port=5
  goalPose : Inport  Port=6
  finalPathPose : Inport  Port=7
  simtime : Inport  Port=8
  curVel : Inport  Port=9
  Enable : EnablePort
  TEBIndexer : Subsystem  TreatAsAtomicUnit=on  VariantControl=TEB Indexer
  TEBMPCCascade : Subsystem  VariantControl=TEB MPC Cascade
  velcmd : Outport
  needLocalReplan : Outport  Port=2
  goalReached : Outport  Port=3
  triggerGlobalReplan : Outport  Port=4
  optcmd : Outport  Port=5
  optposes : Outport  Port=6
  mpcStatus : Outport  Port=7
  nearestIdx : Outport  Port=8
  mpcRefParams : Outport  Port=9

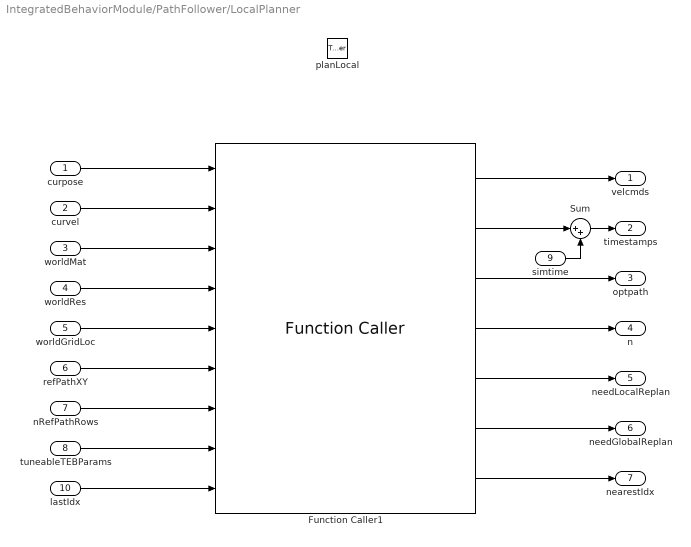
== system IntegratedBehaviorModule/PathFollower/LocalPlanner ==
  curpose : Inport
  curvel : Inport  Port=2
  worldMat : Inport  Port=3
  worldRes : Inport  Port=4
  worldGridLoc : Inport  Port=5
  refPathXY : Inport  Port=6
  nRefPathRows : Inport  Port=7
  tuneableTEBParams : Inport  Port=8
  simtime : Inport  Port=9
  lastIdx : Inport  Port=10
  planLocal : TriggerPort  TriggerType=function-call  VariantControl=(inherit)  PortDimensions=1
  Function Caller1 : FunctionCaller  FunctionPrototype=[velcmds,timestamps,optpath,n,needLocalReplan,needGlobalReplan,nearestIdx] = planLocal(curpose,curvel,worldMat,worldRes,worldGridLoc,refPathXY,nRefPathrows,tuneableTEBParams,lastIdx)  InputArgumentSpecifications=<Enter example>  OutputArgumentSpecifications=<Enter example>
  Sum : Sum  Inputs=|++
  velcmds : Outport
  timestamps : Outport  Port=2
  optpath : Outport  Port=3
  n : Outport  Port=4
  needLocalReplan : Outport  Port=5
  needGlobalReplan : Outport  Port=6
  nearestIdx : Outport  Port=7
  wires:
  worldGridLoc/1 -> Function Caller1/5
  curpose/1 -> Function Caller1/1
  worldMat/1 -> Function Caller1/3
  nRefPathRows/1 -> Function Caller1/7
  Function Caller1/1 -> velcmds/1
  curvel/1 -> Function Caller1/2
  worldRes/1 -> Function Caller1/4
  refPathXY/1 -> Function Caller1/6
  tuneableTEBParams/1 -> Function Caller1/8
  Function Caller1/6 -> needGlobalReplan/1
  Function Caller1/3 -> optpath/1
  Function Caller1/4 -> n/1
  Function Caller1/5 -> needLocalReplan/1
  Function Caller1/2 -> Sum/1
  Sum/1 -> timestamps/1
  simtime/1 -> Sum/2
  Function Caller1/7 -> nearestIdx/1
  lastIdx/1 -> Function Caller1/9

== system IntegratedBehaviorModule/Plant Outputs/Simulink Signals ==
  curpose : Inport
  curvel : Inport  Port=2
  tag scope: curpose=global, curvel=global
  wires:
  curvel/1 -> [curvel]
  curpose/1 -> [curpose]

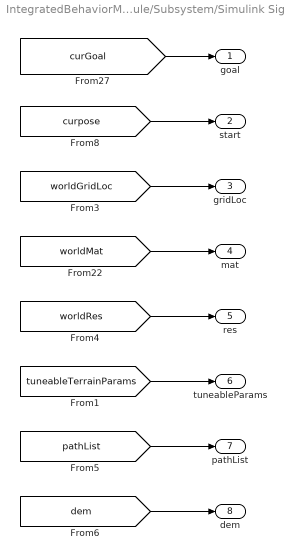
== system IntegratedBehaviorModule/Subsystem/Simulink Signals ==
  goal : Outport
  start : Outport  Port=2
  gridLoc : Outport  Port=3
  mat : Outport  Port=4
  res : Outport  Port=5
  tuneableParams : Outport  Port=6
  pathList : Outport  Port=7
  dem : Outport  Port=8
  wires:
  [tuneableTerrainParams] -> tuneableParams/1
  [worldMat] -> mat/1
  [worldRes] -> res/1
  [dem] -> dem/1
  [pathList] -> pathList/1
  [worldGridLoc] -> gridLoc/1
  [curGoal] -> goal/1
  [curpose] -> start/1

== system IntegratedBehaviorModule/Subsystem1/Simulink Signals ==
  isPlanningRoute : Inport
  isPlanningGlobal : Inport  Port=2
  refPath : Inport  Port=3
  nRefPathRows : Inport  Port=4
  finalPathPose : Inport  Port=5
  tag scope: finalPathPose=global, isPlanningGlobal=global, isPlanningRoute=global, nRefPathRows=global, refPath=global
  wires:
  finalPathPose/1 -> [finalPathPose]
  nRefPathRows/1 -> [nRefPathRows]
  isPlanningRoute/1 -> [isPlanningRoute]
  isPlanningGlobal/1 -> [isPlanningGlobal]
  refPath/1 -> [refPath]

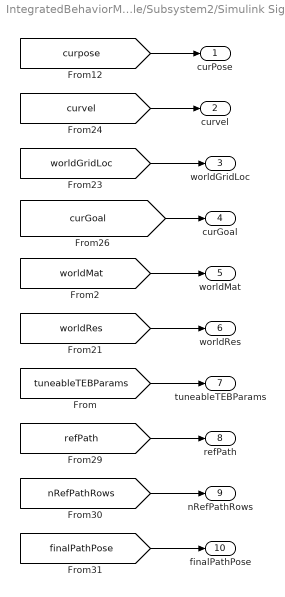
== system IntegratedBehaviorModule/Subsystem2/Simulink Signals ==
  curPose : Outport
  curvel : Outport  Port=2
  worldGridLoc : Outport  Port=3
  curGoal : Outport  Port=4
  worldMat : Outport  Port=5
  worldRes : Outport  Port=6
  tuneableTEBParams : Outport  Port=7
  refPath : Outport  Port=8
  nRefPathRows : Outport  Port=9
  finalPathPose : Outport  Port=10
  wires:
  [worldMat] -> worldMat/1
  [worldGridLoc] -> worldGridLoc/1
  [refPath] -> refPath/1
  [curpose] -> curPose/1
  [tuneableTEBParams] -> tuneableTEBParams/1
  [nRefPathRows] -> nRefPathRows/1
  [finalPathPose] -> finalPathPose/1
  [worldRes] -> worldRes/1
  [curvel] -> curvel/1
  [curGoal] -> curGoal/1

== system IntegratedBehaviorModule/Subsystem3/Simulink Signals ==
  velcmd : Inport
  goalReached : Inport  Port=2
  needLocalReplan : Inport  Port=3
  isPlanningLocal : Inport  Port=4
  needGlobalReplan : Inport  Port=5
  tag scope: hasReachedGoal=global, isPlanningLocal=global, needGlobalReplan=global, needLocalReplan=global, velcmd=global
  wires:
  velcmd/1 -> [velcmd]
  isPlanningLocal/1 -> [isPlanningLocal]
  goalReached/1 -> [hasReachedGoal]
  needGlobalReplan/1 -> [needGlobalReplan]
  needLocalReplan/1 -> [needLocalReplan]

== system IntegratedBehaviorModule/Subsystem4/Simulink Signals ==
  velcmd : Outport
  vehicleParameters : Outport  Port=2
  wires:
  [vehicleParameters] -> vehicleParameters/1
  [velcmd] -> velcmd/1

== system IntegratedBehaviorModule/EnvironmentSensorProcessing/Platform Model/Bicycle Model (2D) ==
  velcmd : Inport
  VehicleParameters : Inport  Port=2
  Bicycle Kinematic Model : robotmobilelib/Bicycle Kinematic Model  VehicleInputs=Vehicle Speed & Heading Angular Velocity  WheelBase=fixedTEBParams.Length  VehicleSpeedRange=[-inf inf]  MaxSteeringAngle=pi/4  InitialState=startPose  SimulateUsing=Interpreted execution
  Demux : Demux  Outputs=2
  Terminator : Terminator
  Terminator1 : Terminator
  curpose : Outport
  curvel : Outport  Port=2
  wires:
  VehicleParameters/1 -> Terminator/1
  velcmd/1 -> curvel/1, Demux/1
  Demux/1 -> Bicycle Kinematic Model/1
  Bicycle Kinematic Model/2 -> Terminator1/1
  Demux/2 -> Bicycle Kinematic Model/2
  Bicycle Kinematic Model/1 -> curpose/1

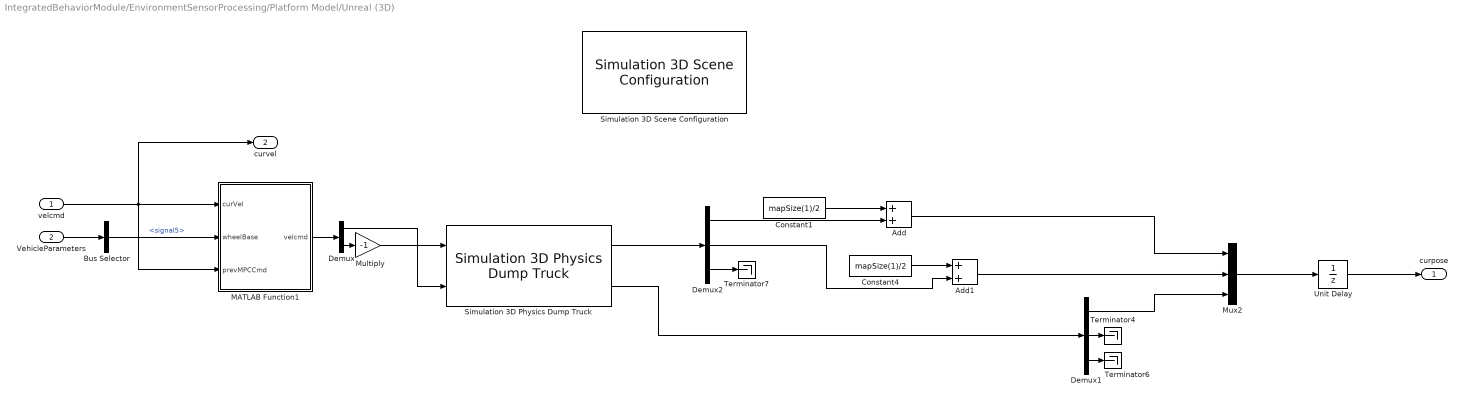
== system IntegratedBehaviorModule/EnvironmentSensorProcessing/Platform Model/Unreal (3D) ==
  velcmd : Inport
  VehicleParameters : Inport  Port=2
  Add : Sum
  Add1 : Sum
  Bus Selector : BusSelector  OutputSignals=signal5
  Constant1 : Constant  Value=mapSize(1)/2  VectorParams1D=off
  Constant4 : Constant  Value=mapSize(1)/2  VectorParams1D=off
  Demux : Demux  Outputs=2
  Demux1 : Demux  Outputs=3
  Demux2 : Demux  Outputs=3
  MATLAB Function1 : MATLAB Function  TreatAsAtomicUnit=on
  Multiply : Gain  Gain=-1
  Mux2 : Mux  Inputs=3
  Simulation 3D Physics Dump Truck : robotsim3dlib/Simulation 3D Physics Dump Truck  TruckType=Standard Dump Truck  TruckColor=Yellow  ActorName=SimulinkVehicle  InitTruckTrans=initialTranslationTruck  InitTruckRot=initialRotationTruck  InitTruckVel=0  InitTruckAccel=0  InitTruckBedAng=0  EnbAccelInp=off  EnbFootBrakInp=off  EnbLifAngInp=off  EnbTruckTransOut=on  EnbTruckRotOut=on  EnbTruckVelOut=off  EnbTruckAngVelOut=off  EnbTruckBedTransOut=off  EnbTruckBedRotOut=off  EnbTruckBedAngOut=off  SampleTime=0.01  ActorType=SimulinkVehicle  ID=C  aMode=6  ActorTag=SimulinkVehicle  Mesh=DumpTruck
  Simulation 3D Scene Configuration : sim3dlib/Simulation 3D Scene Configuration  Priority=0  ProjectFormat=Default Scenes  SceneDesc=Offroad pit mining scene  ProjectName=G:\jobarchive\BR2024ad\2024_03_28_h11m00s59_job2563272_pass\matlab\toolbox\shared\sim3d_projects\automotive_project_windows\UE\WindowsNoEditor\VehicleSimulation.exe  ScenePath=/MathWorksRobotics/Maps/OpenPitMine  EnableOpenDRIVE=off  vehTagList={'Custom';'Scene Origin';'SimulinkVehicle'}  vehTag=Custom  FreeCameraInitialTranslation=initialTranslationTruck([2 1 3]).*[1 -1 1] + [0 0 50]  FreeCameraDefaultInitialTranslation=[-6, 0, 2]  FreeCameraInitialRotation=[0 0 0]  FreeCameraDefaultInitialRotation=[0, -15, 0]  OpVisEn=off  Ts=.02  EnableWindow=on  EnableRemoteAccess=off  EnableWeather=off  SunAzimuth=90  SunAltitude=40.0  EnableGeospatialSun=off  Latitude=0  Longitude=0  Date=2023-01-01  Time=10:30:00  GeoTimeZone=-5.0  SunDaylightSaving=off  wind=1  clouds=10  EnableVolumetricClouds=off  CloudCoverage=0  CloudAltitude=6  fog=0  rain=0  RaindropsEffect=off  SnowDensity=0  EnableGeospatial=off  UseTrueOrigin=off  OriginHeight=200  OriginLatitude=40.744652  OriginLongitude=-73.988864  MapStyle=Aerial  AdditionalAssetIDs=[]  UseAdvancedSunSky=off  SolarTime=11  TimeZone=-5  Day=21  Month=9  Year=2022  UseDaylightSavingTime=on  DSTStartDay=10  DSTStartMonth=3  DSTEndDay=3  DSTEndMonth=11  DSTSwitchHour=2  sensorTag=MainCamera1  sensorId=1  sensorName=MainCamera1  mountLoc=Origin  offsetFlag=off  tmountOffset=[0, 0, 0]  rmountOffset=[0, 0, 0]  HorizontalResolution=1280  VerticalResolution=720  HorizontalFOV=60  mountPoint=[0 0 0]  mountOrientation=[0 0 0]  aMode=5  ID=1  GeoTrigger=Inactive
      settings: LibrarySourceBlock=sl3dlib/Simulation 3D/Environment/Simulation 3D Scene Configuration
  Terminator4 : Terminator
  Terminator6 : Terminator
  Terminator7 : Terminator
  Unit Delay : UnitDelay  SampleTime=-1  HasFrameUpgradeWarning=on
  curpose : Outport
  curvel : Outport  Port=2
  wires:
  Demux2/3 -> Terminator7/1
  Add/1 -> Mux2/1
  Demux1/2 -> Terminator4/1
  velcmd/1 -> MATLAB Function1/3(prevMPCCmd), curvel/1, MATLAB Function1/1(curVel)
  Mux2/1 -> Unit Delay/1
  Demux1/3 -> Terminator6/1
  Demux2/1 -> Add/2
  Constant1/1 -> Add/1
  Simulation 3D Physics Dump Truck/1 -> Demux2/1
  Add1/1 -> Mux2/2
  Demux2/2 -> Add1/2
  Demux1/1 -> Mux2/3
  Constant4/1 -> Add1/1
  Simulation 3D Physics Dump Truck/2 -> Demux1/1
  VehicleParameters/1 -> Bus Selector/1
  Bus Selector/1 -> MATLAB Function1/2(wheelBase)  "<signal5>"
  MATLAB Function1/1(velcmd) -> Demux/1
  Demux/1 -> Simulation 3D Physics Dump Truck/2
  Demux/2 -> Multiply/1
  Multiply/1 -> Simulation 3D Physics Dump Truck/1
  Unit Delay/1 -> curpose/1

== system IntegratedBehaviorModule/Operational Status/Simulink Signals/Confirm New Goal ==
  curGoal : Inport
  Enable : EnablePort
  Display : Display
  NOT : Logic  Operator=NOT  IconShape=distinctive  AllPortsSameDT=off  OutDataTypeStr=boolean
  compareToPrevious : MATLAB Function  TreatAsAtomicUnit=on
  newGoalBlock : Constant  InitFcn=|  Value=goalPose  VectorParams1D=off
      | blockPath = get_param(gcb,'Parent');
      | blockName = get_param(gcb,'Name');
      | 
      | set_param([blockPath '/' blockName],'Value','nan(1,3)')
  isWaiting : Outport
  newGoal : Outport  Port=2
  wires:
  curGoal/1 -> Display/1, compareToPrevious/1(curGoal)
  compareToPrevious/1(isNewGoal) -> NOT/1
  NOT/1 -> isWaiting/1
  newGoalBlock/1 -> newGoal/1, compareToPrevious/2(newGoal)

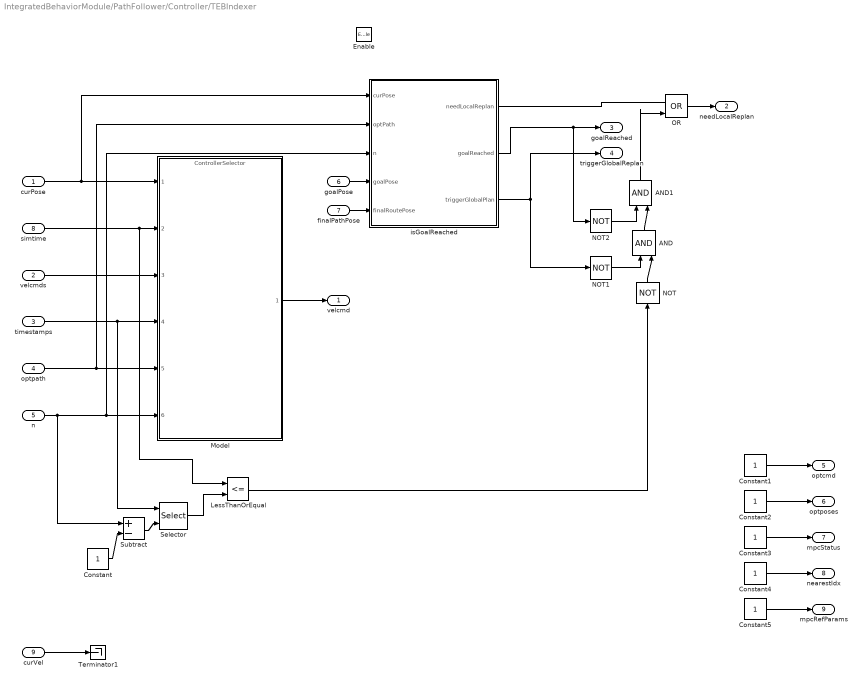
== system IntegratedBehaviorModule/PathFollower/Controller/TEBIndexer ==
  curPose : Inport  PortDimensions=[1 3]
  velcmds : Inport  Port=2
  timestamps : Inport  Port=3
  optpath : Inport  Port=4
  n : Inport  Port=5
  goalPose : Inport  Port=6
  finalPathPose : Inport  Port=7
  simtime : Inport  Port=8
  curVel : Inport  Port=9
  Enable : EnablePort
  AND : Logic  IconShape=distinctive  AllPortsSameDT=off  OutDataTypeStr=boolean
  AND1 : Logic  IconShape=distinctive  AllPortsSameDT=off  OutDataTypeStr=boolean
  Constant{,1..5} (6 alike) : Constant
  LessThanOrEqual : RelationalOperator  Operator=<=  OutDataTypeStr=boolean  RndMeth=Simplest  InputSameDT=off
  Model : ModelReference  ModelNameDialog=ControllerSelector.slx  SimulationMode=Normal  ModelReferenceVersion=1.1
  NOT : Logic  Operator=NOT  IconShape=distinctive  AllPortsSameDT=off  OutDataTypeStr=boolean
  NOT1 : Logic  Operator=NOT  IconShape=distinctive  AllPortsSameDT=off  OutDataTypeStr=boolean
  NOT2 : Logic  Operator=NOT  IconShape=distinctive  AllPortsSameDT=off  OutDataTypeStr=boolean
  OR : Logic  Operator=OR  IconShape=distinctive  AllPortsSameDT=off  OutDataTypeStr=boolean
  Selector : Selector  NumberOfDimensions=2  InputPortWidth=1  IndexOptions=Index vector (port),Select all  Indices=[1 3],1  OutputSizes=1,1
  Subtract : Sum  Inputs=+-
  Terminator1 : Terminator
  isGoalReached : Subsystem
  velcmd : Outport  OutputWhenDisabled=reset  InitialOutput=[0 0]
  needLocalReplan : Outport  Port=2
  goalReached : Outport  Port=3
  triggerGlobalReplan : Outport  Port=4  OutputWhenDisabled=reset  InitialOutput=0
  optcmd : Outport  Port=5
  optposes : Outport  Port=6
  mpcStatus : Outport  Port=7
  nearestIdx : Outport  Port=8
  mpcRefParams : Outport  Port=9
  wires:
  simtime/1 -> LessThanOrEqual/1, Model/2
  velcmds/1 -> Model/3
  timestamps/1 -> Selector/1, Model/4
  optpath/1 -> isGoalReached/2(optPath), Model/5
  n/1 -> Subtract/1, isGoalReached/3(n), Model/6
  Model/1 -> velcmd/1
  Selector/1 -> LessThanOrEqual/2
  LessThanOrEqual/1 -> NOT/1
  curPose/1 -> Model/1, isGoalReached/1(curPose)
  isGoalReached/1(needLocalReplan) -> OR/1
  isGoalReached/2(goalReached) -> goalReached/1, NOT2/1
  goalPose/1 -> isGoalReached/4(goalPose)
  Constant/1 -> Subtract/2
  Subtract/1 -> Selector/2
  OR/1 -> needLocalReplan/1
  NOT/1 -> AND/2
  isGoalReached/3(triggerGlobalPlan) -> NOT1/1, triggerGlobalReplan/1
  finalPathPose/1 -> isGoalReached/5(finalRoutePose)
  AND/1 -> AND1/2
  NOT1/1 -> AND/1
  NOT2/1 -> AND1/1
  AND1/1 -> OR/2
  curVel/1 -> Terminator1/1
  Constant1/1 -> optcmd/1
  Constant2/1 -> optposes/1
  Constant3/1 -> mpcStatus/1
  Constant4/1 -> nearestIdx/1
  Constant5/1 -> mpcRefParams/1

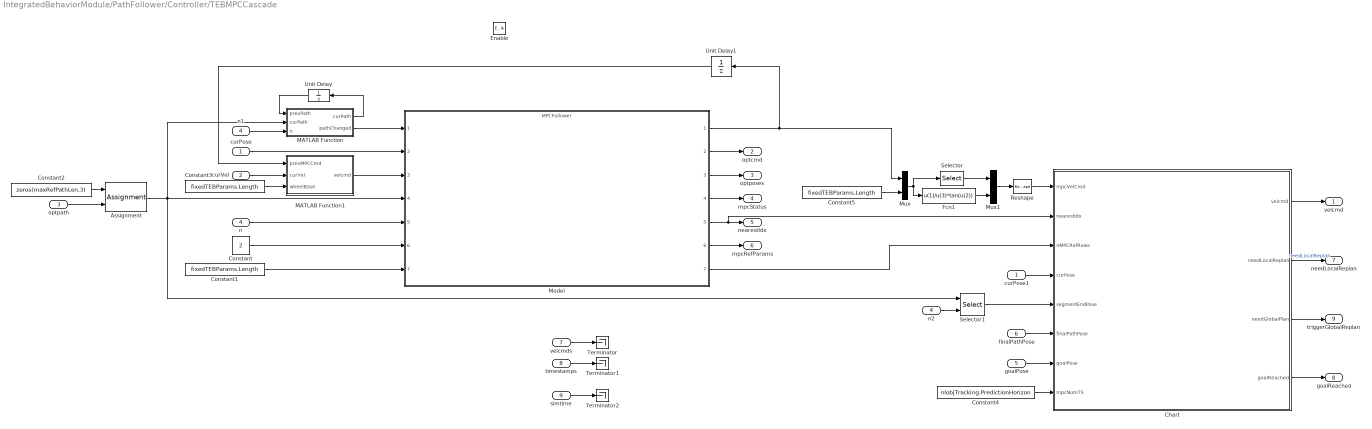
== system IntegratedBehaviorModule/PathFollower/Controller/TEBMPCCascade ==
  curPose : Inport  SampleTime=nlobjTracking.Ts
  curVel : Inport  Port=2  SampleTime=nlobjTracking.Ts
  optpath : Inport  Port=3  SampleTime=nlobjTracking.Ts
  n : Inport  Port=4  SampleTime=nlobjTracking.Ts
  goalPose : Inport  Port=5
  finalPathPose : Inport  Port=6
  velcmds : Inport  Port=7
  timestamps : Inport  Port=8
  simtime : Inport  Port=9
  Enable : EnablePort
  Assignment : Assignment  NumberOfDimensions=2  DiagnosticForDimensions=Warning  IndexOptions=Starting index (dialog),Starting index (dialog)  Indices=1,1  OutputSizes=1,1
  Chart : Stateflow chart  TreatAsAtomicUnit=on
      settings: PortSchema="{\"entries\":[{\"content\":{\"sides\":[{\"content\":{\"connectorIds\":[\"In8\",\"In2\",\"In1\",\"In4\",\"In5\",\"In6\",\"In7\",\"In3\"]},\"type\":\"ConnectorPlacement.EquallySpacedRectSide\",\"uuid\":\"08395831-dbae-49cf-844d-729862efb56c\"},{\"content\":{\"connectorIds\":[\"Out4\",\"Out1\",\"Out2\",\"Out3\"],\"side\":\"RIGHT\"},\"type\":\"ConnectorPlacement.EquallySpacedRectSide\",\"uuid\":\"7aab2f4b-f147-41f5-84a6-1ccf26292ffc\"},{\"content\":{\"side\":\"TOP\"},\"type\":\"ConnectorPlacement.EquallySpacedRectSide\",\"uuid\":\"fd7335e6-a9e8-4ff2-a346-83748e189f04\"}]},\"type\":\"ConnectorPlacement.EquallySpacedConnector\",\"uuid\":\"68ab2c9d-d2a2-4341-98a3-3a3d7759d72e\"}],\"packageUris\":[\"http://schema.mathworks.com/mf0/Connector/R2020b\"],\"version\":\"1.0\"}"
  Constant : Constant  Value=2
  Constant1 : Constant  Value=fixedTEBParams.Length
  Constant2 : Constant  Value=zeros(maxRefPathLen,3)
  Constant3 : Constant  Value=fixedTEBParams.Length
  Constant4 : Constant  Value=nlobjTracking.PredictionHorizon
  Constant5 : Constant  Value=fixedTEBParams.Length
  Fcn1 : Fcn  Expr=u(1)/u(3)*tan(u(2))
  MATLAB Function : MATLAB Function  TreatAsAtomicUnit=on
  MATLAB Function1 : MATLAB Function  TreatAsAtomicUnit=on
  Model : ModelReference  ModelNameDialog=MPCFollower.slx  SimulationMode=Normal  ModelReferenceVersion=1.2
  Mux : Mux  Inputs=2
  Mux1 : Mux  Inputs=2
  Reshape : Reshape  OutputDimensionality=Row vector (2-D)
  Selector : Selector  InputPortWidth=3  IndexOptions=Index vector (dialog)  Indices=1  OutputSizes=1
  Selector1 : Selector  NumberOfDimensions=2  InputPortWidth=3  IndexOptions=Index vector (port),Select all  Indices=[1 3],1  OutputSizes=1,1
  Terminator : Terminator
  Terminator1 : Terminator
  Terminator2 : Terminator
  Unit Delay : UnitDelay  SampleTime=-1  HasFrameUpgradeWarning=on
  Unit Delay1 : UnitDelay  SampleTime=-1  HasFrameUpgradeWarning=on
  curPose1 : InportShadow  SampleTime=nlobjTracking.Ts
  n1 : InportShadow  Port=4  SampleTime=nlobjTracking.Ts
  n2 : InportShadow  Port=4  SampleTime=nlobjTracking.Ts
  velcmd : Outport
  optcmd : Outport  Port=2
  optposes : Outport  Port=3
  mpcStatus : Outport  Port=4
  nearestIdx : Outport  Port=5
  mpcRefParams : Outport  Port=6
  needLocalReplan : Outport  Port=7  OutputWhenDisabled=reset  InitialOutput=0
  goalReached : Outport  Port=8  OutputWhenDisabled=reset  InitialOutput=0
  triggerGlobalReplan : Outport  Port=9  OutputWhenDisabled=reset  InitialOutput=0
  wires:
  Chart/2(needGlobalPlan) -> triggerGlobalReplan/1
  Model/2 -> optcmd/1
  Chart/3(goalReached) -> goalReached/1
  Constant1/1 -> Model/7
  Constant/1 -> Model/6
  finalPathPose/1 -> Chart/6(finalPathPose)
  Model/6 -> mpcRefParams/1
  goalPose/1 -> Chart/7(goalPose)
  curVel/1 -> MATLAB Function1/2(curVel)
  optpath/1 -> Assignment/2
  Model/3 -> optposes/1
  Model/4 -> mpcStatus/1
  Model/5 -> Chart/2(nearestIdx), nearestIdx/1
  velcmds/1 -> Terminator/1
  timestamps/1 -> Terminator1/1
  simtime/1 -> Terminator2/1
  Constant2/1 -> Assignment/1
  Model/7 -> Chart/1(nMPCRefRows)
  Fcn1/1 -> Mux1/2
  Selector/1 -> Mux1/1
  Mux/1 -> Selector/1, Fcn1/1
  Model/1 -> Unit Delay1/1, Mux/1
  Unit Delay1/1 -> MATLAB Function1/1(prevMPCCmd)
  Constant4/1 -> Chart/3(mpcNumTS)
  Selector1/1 -> Chart/5(segmentEndPose)
  Chart/4(velcmd) -> velcmd/1
  Chart/1(needLocalReplan) -> needLocalReplan/1  "needLocalReplan"
  Mux1/1 -> Reshape/1
  Reshape/1 -> Chart/8(mpcVelCmd)
  MATLAB Function/2(pathChanged) -> Model/1
  Assignment/1 -> Model/4, MATLAB Function/2("curPath "), Selector1/1
  MATLAB Function/1(curPath) -> Unit Delay/1
  Unit Delay/1 -> MATLAB Function/1(prevPath)
  curPose/1 -> Model/2
  MATLAB Function1/1(velcmd) -> Model/3
  curPose1/1 -> Chart/4(curPose)
  n1/1 -> MATLAB Function/3(n)
  n2/1 -> Selector1/2
  n/1 -> Model/5
  Constant3/1 -> MATLAB Function1/3(wheelBase)
  Constant5/1 -> Mux/2
